simulink model "Cinematica_Inversa_Jacobiana_Pseudoinversa"  (R2015a)
settings: Solver=ode45  StartTime=0.0  StopTime=2  FixedStep=0.001  RelTol=1e-3
values from neighbouring files (symbols this model uses):
  dif_t = in(9)    [Euler.m]    (also in rob_sic.m = 0.001)
settings Model: Creator=TRIANOSAURIO  LastModifiedBy=TRIANOSAURIO
settings ConfigComp: CovMetricSettings=dw  CovHtmlReporting=on  CovSaveCumulativeToWorkspaceVar=on  CovSaveSingleToWorkspaceVar=on  CovExternalEMLEnable=off

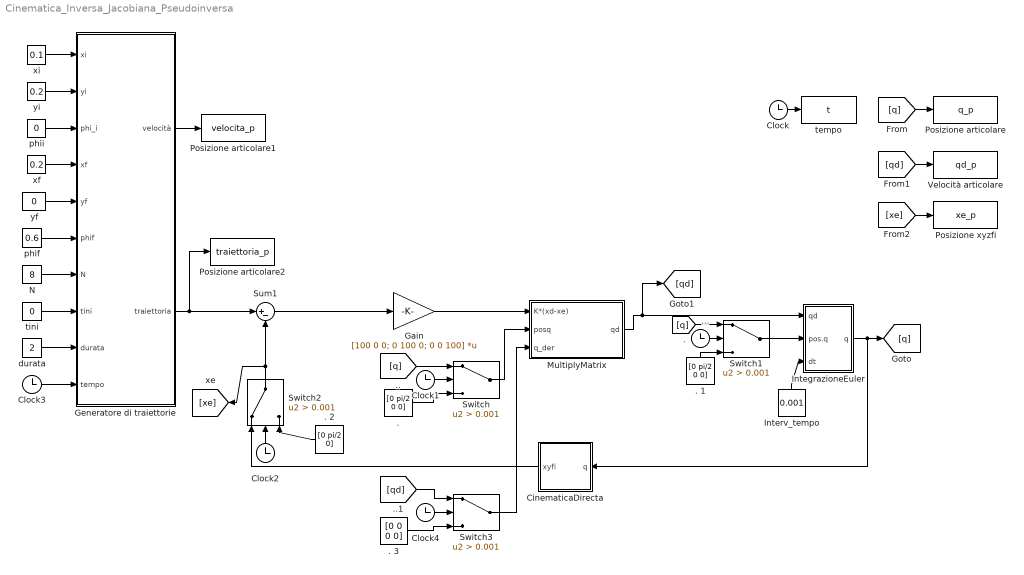
== system Cinematica_Inversa_Jacobiana_Pseudoinversa ==
  ". " : Constant  Value=[0 pi/2 0 0]
  . 1 : Constant  Value=[0 pi/2 0 0]
  . 2 : Constant  Value=[0 pi/2 0]
  . 3 : Constant  Value=[0 0 0 0]
  "... " : Clock
  CinematicaDirecta : Subsystem
  Clock{,1..4} (5 alike) : Clock
  Gain : Gain  Gain=[100 0 0; 0 100 0; 0 0 100]  Multiplication=Matrix(K*u)
  Generatore di traiettorie : Subsystem
  IntegrazioneEuler : Subsystem
  Interv_tempo : Constant  Value=0.001
  MultiplyMatrix : Subsystem
  N : Constant  Value=8
  Posizione articolare : ToWorkspace  VariableName=q_p  SampleTime=dif_t
  Posizione articolare1 : ToWorkspace  VariableName=velocita_p  SampleTime=dif_t
  Posizione articolare2 : ToWorkspace  VariableName=traiettoria_p  SampleTime=dif_t
  "Posizione xyzfi " : ToWorkspace  VariableName=xe_p  SampleTime=dif_t
  Sum1 : Sum  Inputs=|+-
  Switch{,1..3} (4 alike) : Switch  Criteria=u2 > Threshold  Threshold=0.001
  Velocità articolare : ToWorkspace  VariableName=qd_p  SampleTime=dif_t
  durata : Constant  Value=2
  phif : Constant  Value=0.6
  phii : Constant  Value=0
  tempo : ToWorkspace  VariableName=t  SampleTime=0.001
  tini : Constant  Value=0
  xf : Constant  Value=0.2
  xi : Constant  Value=0.1
  yf : Constant  Value=0
  yi : Constant  Value=0.2
  wires:
  Sum1/1 -> Gain/1
  Clock/1 -> tempo/1
  IntegrazioneEuler/1(q) -> CinematicaDirecta/1(q), [q]
  [q] -> Posizione articolare/1
  Gain/1 -> MultiplyMatrix/1(K*(xd-xe))
  Interv_tempo/1 -> IntegrazioneEuler/3(dt)
  Switch/1 -> MultiplyMatrix/2(posq)
  Clock1/1 -> Switch/2
  [q] -> Switch1/1
  Switch1/1 -> IntegrazioneEuler/2(pos.q)
  "... "/1 -> Switch1/2
  . 1/1 -> Switch1/3
  [q] -> Switch/1
  ". "/1 -> Switch/3
  Switch2/1 -> Sum1/2, [xe]
  CinematicaDirecta/1(xyfi) -> Switch2/1
  Clock2/1 -> Switch2/2
  . 2/1 -> Switch2/3
  [qd] -> Velocità articolare/1
  [xe] -> "Posizione xyzfi "/1
  xi/1 -> Generatore di traiettorie/1(xi)
  yi/1 -> Generatore di traiettorie/2(yi)
  phii/1 -> Generatore di traiettorie/3(phi_i)
  xf/1 -> Generatore di traiettorie/4(xf)
  yf/1 -> Generatore di traiettorie/5(yf)
  tini/1 -> Generatore di traiettorie/8(tini)
  durata/1 -> Generatore di traiettorie/9(durata)
  Clock3/1 -> Generatore di traiettorie/10(tempo)
  Generatore di traiettorie/2("traiettoria ") -> Sum1/1, Posizione articolare2/1
  Generatore di traiettorie/1(velocità) -> Posizione articolare1/1
  MultiplyMatrix/1(qd) -> [qd], IntegrazioneEuler/1(qd)
  . 3/1 -> Switch3/3
  [qd] -> Switch3/1
  Clock4/1 -> Switch3/2
  Switch3/1 -> MultiplyMatrix/3(q_der)
  N/1 -> Generatore di traiettorie/7(N)
  phif/1 -> Generatore di traiettorie/6(phif)

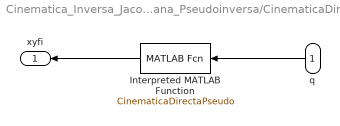
== system Cinematica_Inversa_Jacobiana_Pseudoinversa/CinematicaDirecta ==
  q : Inport
  Interpreted MATLAB Function : MATLABFcn  MATLABFcn=CinematicaDirectaPseudo  OutputDimensions=3
  xyfi : Outport
  wires:
  q/1 -> Interpreted MATLAB Function/1
  Interpreted MATLAB Function/1 -> xyfi/1

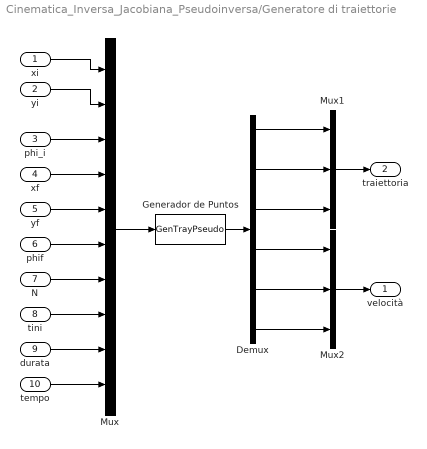
== system Cinematica_Inversa_Jacobiana_Pseudoinversa/Generatore di traiettorie ==
  xi : Inport
  yi : Inport  Port=2
  phi_i : Inport  Port=3
  xf : Inport  Port=4
  yf : Inport  Port=5
  phif : Inport  Port=6
  N : Inport  Port=7
  tini : Inport  Port=8
  durata : Inport  Port=9
  tempo : Inport  Port=10
  Demux : Demux  Outputs=6
  Generador de Puntos : MATLABFcn  MATLABFcn=GenTrayPseudo  OutputDimensions=6
  Mux : Mux  Inputs=10
  Mux1 : Mux  Inputs=3
  Mux2 : Mux  Inputs=3
  velocità : Outport
  "traiettoria " : Outport  Port=2
  wires:
  Mux/1 -> Generador de Puntos/1
  xi/1 -> Mux/1
  yi/1 -> Mux/2
  Generador de Puntos/1 -> Demux/1
  Mux1/1 -> "traiettoria "/1
  Mux2/1 -> velocità/1
  phi_i/1 -> Mux/3
  xf/1 -> Mux/4
  yf/1 -> Mux/5
  phif/1 -> Mux/6
  N/1 -> Mux/7
  tini/1 -> Mux/8
  durata/1 -> Mux/9
  tempo/1 -> Mux/10
  Demux/4 -> Mux2/1
  Demux/5 -> Mux2/2
  Demux/6 -> Mux2/3
  Demux/3 -> Mux1/3
  Demux/2 -> Mux1/2
  Demux/1 -> Mux1/1

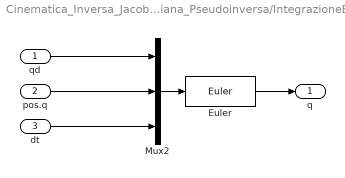
== system Cinematica_Inversa_Jacobiana_Pseudoinversa/IntegrazioneEuler ==
  qd : Inport
  pos.q : Inport  Port=2
  dt : Inport  Port=3
  Euler : MATLABFcn  MATLABFcn=Euler
  Mux2 : Mux  Inputs=3
  q : Outport
  wires:
  Euler/1 -> q/1
  qd/1 -> Mux2/1
  Mux2/1 -> Euler/1
  pos.q/1 -> Mux2/2
  dt/1 -> Mux2/3

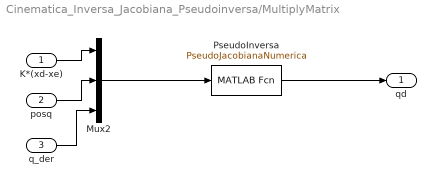
== system Cinematica_Inversa_Jacobiana_Pseudoinversa/MultiplyMatrix ==
  K*(xd-xe) : Inport
  posq : Inport  Port=2
  q_der : Inport  Port=3
  Mux2 : Mux  Inputs=3
  "PseudoInversa " : MATLABFcn  MATLABFcn=PseudoJacobianaNumerica
  qd : Outport
  wires:
  "PseudoInversa "/1 -> qd/1
  Mux2/1 -> "PseudoInversa "/1
  K*(xd-xe)/1 -> Mux2/1
  posq/1 -> Mux2/2
  q_der/1 -> Mux2/3
